simulink model "integrated_model"  (R2020b)
settings: Solver=VariableStepAuto  StartTime=0.0  StopTime=10  RelTol=1e-3
undefined symbols (not defined in the file): sigbuilder_block
settings Model: Creator=Training  LastModifiedBy=Training

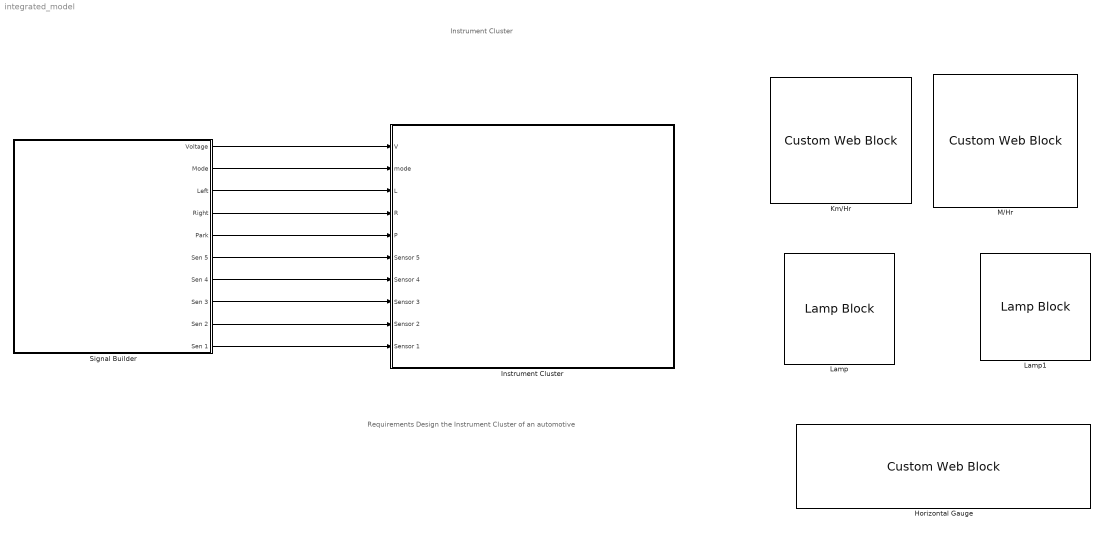
== system integrated_model ==
  note: Requirements
      | Design the Instrument Cluster of an automotive
  note: Instrument Cluster
  Horizontal Gauge : CustomWebBlock  ShowInitialText=on  Configuration="{\"components\":[{\"name\":\"LinearScaleComponent\",\"settings\":{\"bounds\":{\"max\":5,\"min\":0,\"tickInterval\":\"auto\"},\"internalTickHeightScaleFactor\":0.5,\"labelColor\":[250,245,199],\"labelFont\":{\"font\":\"Arial\",\"fontSize\":12},\"labelTransparency\":1,\"needleImage\":{\"size\":[21,75],\"src\":\"data:image\\/svg+xml;base64,PHN2ZyB4bWxucz0iaHR0cDovL3d3dy53My5vcmcvMjAwMC9zdmciIHhtbG5zOnhsaW5rPSJodHRwOi8vd3d3LnczLm9yZy8xOTk5L3hsaW5rIiB2aWV3Qm94PSIwIDAgMjEgNzUiPjxkZWZzPjxzdHlsZT4uY2xzLTF7ZmlsbDpub25lO30uY2xzLTJ7aXNvbGF0aW9uOmlzb2xhdGU7fS5jbHMtM3tjbGlwLXBhdGg6dXJsKCNjbGlwLXBhdGgpO30uY2xzLTR7b3BhY2l0eTowLjM7bWl4LWJsZW5kLW1vZGU6bXVsdGlwbHk7fS5jbHMtNXtmaWxsOiNlYjI2Mjk7fTwvc3R5bGU+PGNsaXBQYXRoIGlkPSJjbGlwLXBhdGgiIHRyYW5zZm9y ...(+1928 chars)\",\"srcOrientation\":\"horizontal\"},\"needleOffset\":[0,0.01094391244870041],\"needleSize\":{\"height\":0.7589285714285714,\"width\":0.11960078534031414},\"position\":[0.06986607142857143,0.01995798319327731,0.9641544117647058,0.8],\"scaleColors\":[],\"scaleColorsSize\":0.2,\"showLabels\":1,\"showMinorTicks\":0,\"showSpanLine\":1,\"showTicks\":1,\"tickColor\":[250,245,200],\"tickTransparency\":1,\"valueBarColor\":[23,89,176],\"valueBarOffset\":0,\"valueBarSize\":0.23,\"valueBarTransparency\":1}},{\"name\":\"BackgroundImageComponent\",\"settings\":{\"image\":{\"size\":[380,101],\"src\":\"data:image\\/svg+xml;base64,PHN2ZyB4bWxucz0iaHR0cDovL3d3dy53My5vcmcvMjAwMC9zdmciIHZpZXdCb3g9IjAgMCAzODAgMTAxIj48ZGVmcz48c3R5bGU+LmNscy0xe2ZpbGw6IzAwMmI0Mjt9LmNscy0ye2ZpbGw6IzQyNzA4Mjt9LmNscy0ze2ZpbGw6IzdjYTBiMjt9PC9zdHlsZT48L2RlZnM+PHRpdGxlPmhvcml6b250YWxfZ2F1Z2VfIGJhY2tncm91bmQ8L3RpdGxlPjxnIGlkPSJMYXllcl8yIiBkYXRhLW5hbWU9IkxheWVyIDIiPjxnIGlkPSJMYXllcl8xLTIiIGRhdGEtbmFtZT0iTGF5ZXIgMSI+PHJlY3QgY2xhc3M9ImNscy0xIiB4PSIxMSIgeT0iMTEiIHdpZHRoPSIzNTgiIGhlaWdodD0iNzkiLz48cGF0aCBjbGFzcz0iY2xzLTIiIGQ9Ik04LDhWOTNIMzcyVjhaTTM2OSw5MEgxMVYxMUgzNjlaIi8+PHBhdGggY2xhc3M9ImNscy0zIiBkPSJNMCwwVjEwMUgzODBWMFpNMzcyLDkzSDhWOEgzNzJaIi8+PC9nPjwvZz48L3N2Zz4=\",\"srcOrientation\":\"horizontal\"},\"position\":[0,0,1,1],\"scaleMode\":\"0\"}},{\"name\":\"ForegroundImageComponent\",\"settings\":{\"image\":{\"size\":[0,0],\"src\":\"default\",\"srcOrientation\":[]},\"isForeground\":1,\"position\":[0,0,1,1],\"scaleMode\":\"0\"}}],\"settings\":{\"BindingType\":\"signal\",\"aspectRatio\":3.8,\"fixedAspectRatio\":\"on\",\"orientation\":\"horizontal\"},\"type\":\"LinearGauge\"}"
  Instrument Cluster : Subsystem
  Km/Hr : CustomWebBlock  LabelPosition=Hide  ShowInitialText=on  Configuration="{\"components\":[{\"name\":\"CircularScaleComponent\",\"settings\":{\"bounds\":{\"max\":100,\"min\":0,\"tickInterval\":\"auto\"},\"direction\":\"cw\",\"flipLimits\":0,\"innerRadius\":0.75,\"internalTickHeightScaleFactor\":1,\"labelColor\":[255,252,199],\"labelFont\":{\"font\":\"Arial\",\"fontSize\":12},\"labelTransparency\":1,\"minorTickHeightScaleFactor\":0.2,\"needleImage\":{\"size\":[1890,567],\"src\":\"data:image\\/svg+xml;base64,PD94bWwgdmVyc2lvbj0iMS4wIiBlbmNvZGluZz0iVVRGLTgiIHN0YW5kYWxvbmU9Im5vIj8+CjxzdmcKICAgeG1sbnM6ZGM9Imh0dHA6Ly9wdXJsLm9yZy9kYy9lbGVtZW50cy8xLjEvIgogICB4bWxuczpjYz0iaHR0cDovL2NyZWF0aXZlY29tbW9ucy5vcmcvbnMjIgogICB4bWxuczpyZGY9Imh0dHA6Ly93d3cudzMub3JnLzE5OTkvMDIvMjItcmRmLXN5bnRheC1ucyMiCiAgIHhtbG5zOnN2Zz0iaHR0cDovL3d3dy53My5vcmcvMjAwMC9zdmciCiAgIHhtbG5zPSJodHRwOi8vd3d3LnczLm9yZy8yMDAwL3N2ZyIKICAgeG1sbnM6 ...(+4096 chars)\"},\"needleOffset\":[0.1610917094974375,0],\"needleOrientation\":-45,\"needleRotation\":180.59702388394928,\"needleSize\":{\"height\":0.13032601008944536,\"width\":0.416859542883425},\"outerRadius\":0.9,\"position\":[0.06486742424242424,0.05627705627705628,0.8917748917748918,0.8787878787878788],\"scaleAngle\":270,\"scaleAngleOffset\":135,\"scaleColors\":[],\"scaleColorsSize\":0.2,\"scalePosition\":[0,0,1,1],\"showLabels\":1,\"showMinorTicks\":1,\"showSpanLine\":1,\"showTicks\":1,\"tickColor\":[15,255,255],\"tickTransparency\":1,\"valueBarColor\":[19,159,255],\"valueBarPosition\":[0,0,1,1],\"valueBarSize\":0.2,\"valueBarTransparency\":1}},{\"name\":\"BackgroundImageComponent\",\"settings\":{\"image\":{\"size\":[500,500],\"src\":\"data:image\\/svg+xml;base64,PD94bWwgdmVyc2lvbj0iMS4wIiBlbmNvZGluZz0iVVRGLTgiIHN0YW5kYWxvbmU9Im5vIj8+CjxzdmcKICAgeG1sbnM6ZGM9Imh0dHA6Ly9wdXJsLm9yZy9kYy9lbGVtZW50cy8xLjEvIgogICB4bWxuczpjYz0iaHR0cDovL2NyZWF0aXZlY29tbW9ucy5vcmcvbnMjIgogICB4bWxuczpyZGY9Imh0dHA6Ly93d3cudzMub3JnLzE5OTkvMDIvMjItcmRmLXN5bnRheC1ucyMiCiAgIHhtbG5zOnN2Zz0iaHR0cDovL3d3dy53My5vcmcvMjAwMC9zdmciCiAgIHhtbG5zPSJodHRwOi8vd3d3LnczLm9yZy8yMDAwL3N2ZyIKICAgeG1sbnM6 ...(+9964 chars)\"},\"position\":[0,0,1,1],\"scaleMode\":\"0\"}},{\"name\":\"ForegroundImageComponent\",\"settings\":{\"image\":{\"size\":[0,0],\"src\":\"default\",\"srcOrientation\":[]},\"isForeground\":1,\"position\":[0,0,1,1],\"scaleMode\":\"0\"}}],\"settings\":{\"BindingType\":\"signal\",\"aspectRatio\":1.035294117647059,\"direction\":\"cw\",\"fixedAspectRatio\":\"on\",\"flipLimits\":0,\"orientation\":\"horizontal\"},\"type\":\"CircularGauge\"}"
  Lamp : LampBlock
  Lamp1 : LampBlock
  M/Hr : CustomWebBlock  LabelPosition=Hide  ShowInitialText=on  Configuration="{\"components\":[{\"name\":\"CircularScaleComponent\",\"settings\":{\"bounds\":{\"max\":100,\"min\":0,\"tickInterval\":\"auto\"},\"direction\":\"cw\",\"flipLimits\":0,\"innerRadius\":0.75,\"internalTickHeightScaleFactor\":1,\"labelColor\":[0,114,189],\"labelFont\":{\"font\":\"Arial\",\"fontSize\":12},\"labelTransparency\":1,\"minorTickHeightScaleFactor\":0.2,\"needleImage\":{\"size\":[1890,567],\"src\":\"data:image\\/svg+xml;base64,PD94bWwgdmVyc2lvbj0iMS4wIiBlbmNvZGluZz0iVVRGLTgiIHN0YW5kYWxvbmU9Im5vIj8+CjxzdmcKICAgeG1sbnM6ZGM9Imh0dHA6Ly9wdXJsLm9yZy9kYy9lbGVtZW50cy8xLjEvIgogICB4bWxuczpjYz0iaHR0cDovL2NyZWF0aXZlY29tbW9ucy5vcmcvbnMjIgogICB4bWxuczpyZGY9Imh0dHA6Ly93d3cudzMub3JnLzE5OTkvMDIvMjItcmRmLXN5bnRheC1ucyMiCiAgIHhtbG5zOnN2Zz0iaHR0cDovL3d3dy53My5vcmcvMjAwMC9zdmciCiAgIHhtbG5zPSJodHRwOi8vd3d3LnczLm9yZy8yMDAwL3N2ZyIKICAgeG1sbnM6 ...(+4096 chars)\"},\"needleOffset\":[0.1610917094974375,0],\"needleOrientation\":-45,\"needleRotation\":180.59702388394928,\"needleSize\":{\"height\":0.13032601008944536,\"width\":0.416859542883425},\"outerRadius\":0.9,\"position\":[0.06475601604278075,0.05626539408866995,0.8917795566502463,0.8787600267379679],\"scaleAngle\":270,\"scaleAngleOffset\":135,\"scaleColors\":[],\"scaleColorsSize\":0.2,\"scalePosition\":[0,0,1,1],\"showLabels\":1,\"showMinorTicks\":1,\"showSpanLine\":1,\"showTicks\":1,\"tickColor\":[100,212,19],\"tickTransparency\":1,\"valueBarColor\":[0,114,189],\"valueBarPosition\":[0,0,1,1],\"valueBarSize\":0.2,\"valueBarTransparency\":1}},{\"name\":\"BackgroundImageComponent\",\"settings\":{\"image\":{\"size\":[500,500],\"src\":\"data:image\\/svg+xml;base64,PD94bWwgdmVyc2lvbj0iMS4wIiBlbmNvZGluZz0iVVRGLTgiIHN0YW5kYWxvbmU9Im5vIj8+CjxzdmcKICAgeG1sbnM6ZGM9Imh0dHA6Ly9wdXJsLm9yZy9kYy9lbGVtZW50cy8xLjEvIgogICB4bWxuczpjYz0iaHR0cDovL2NyZWF0aXZlY29tbW9ucy5vcmcvbnMjIgogICB4bWxuczpyZGY9Imh0dHA6Ly93d3cudzMub3JnLzE5OTkvMDIvMjItcmRmLXN5bnRheC1ucyMiCiAgIHhtbG5zOnN2Zz0iaHR0cDovL3d3dy53My5vcmcvMjAwMC9zdmciCiAgIHhtbG5zPSJodHRwOi8vd3d3LnczLm9yZy8yMDAwL3N2ZyIKICAgeG1sbnM6 ...(+9964 chars)\"},\"position\":[0,0,1,1],\"scaleMode\":\"0\"}},{\"name\":\"ForegroundImageComponent\",\"settings\":{\"image\":{\"size\":[0,0],\"src\":\"default\",\"srcOrientation\":[]},\"isForeground\":1,\"position\":[0,0,1,1],\"scaleMode\":\"0\"}}],\"settings\":{\"BindingType\":\"signal\",\"aspectRatio\":1.085561497326203,\"direction\":\"cw\",\"fixedAspectRatio\":\"on\",\"flipLimits\":0,\"orientation\":\"horizontal\"},\"type\":\"CircularGauge\"}"
  Signal Builder : Subsystem  Tag=STV Subsys  LoadFcn=sigbuilder_block('load');  StartFcn=sigbuilder_block('start');  StopFcn=sigbuilder_block('stop');  ClipboardFcn=sigbuilder_block('clipboard');  mask(Sigbuilder block){tuvar=[0:10]}
      mask help: Simulink:masks:SigbuilderBlock_MD
      mask init:
      | if ~strcmp(get_param(bdroot(gcbh),'SimulationStatus'),'stopped') tuvar = sigbuilder_block('maskInit'); end
      settings: CopyFcn=sigbuilder_block('copy');  DeleteFcn=sigbuilder_block('delete');  ModelCloseFcn=sigbuilder_block('modelClose');  PreSaveFcn=sigbuilder_block('preSave');  PauseFcn=sigbuilder_block('pause');  ContinueFcn=sigbuilder_block('continue');  NameChangeFcn=sigbuilder_block('namechange');  OpenFcn=sigbuilder_block('open',[539.25 204.75 550.5 399.75 ]);  CloseFcn=sigbuilder_block('close');
      mask Display: plot(0, 0, 100, 100,[2, 2, 32, 32, 2], [68, 8, 8, 68, 68],[32, 2], [38, 38], [32, 19, 2],[53, 60, 44], [32, 17, 17, 2],[16, 16, 31, 31]);txt = getActiveGroup(gcbh);text(2, 100, txt,'verticalAlignment', 'top');
  wires:
  Signal Builder/1(Voltage) -> Instrument Cluster/1(V)
  Signal Builder/2(Mode) -> Instrument Cluster/2(mode)
  Signal Builder/3(Left) -> Instrument Cluster/3(L)
  Signal Builder/4(Right) -> Instrument Cluster/4(R)
  Signal Builder/5(Park) -> Instrument Cluster/5(P)
  Signal Builder/6("Sen 5 ") -> Instrument Cluster/6(Sensor 5)
  Signal Builder/7(Sen 4) -> Instrument Cluster/7(Sensor 4)
  Signal Builder/8(Sen 3) -> Instrument Cluster/8(Sensor 3)
  Signal Builder/9(" Sen 2") -> Instrument Cluster/9(Sensor 2)
  Signal Builder/10(Sen 1) -> Instrument Cluster/10(Sensor 1)

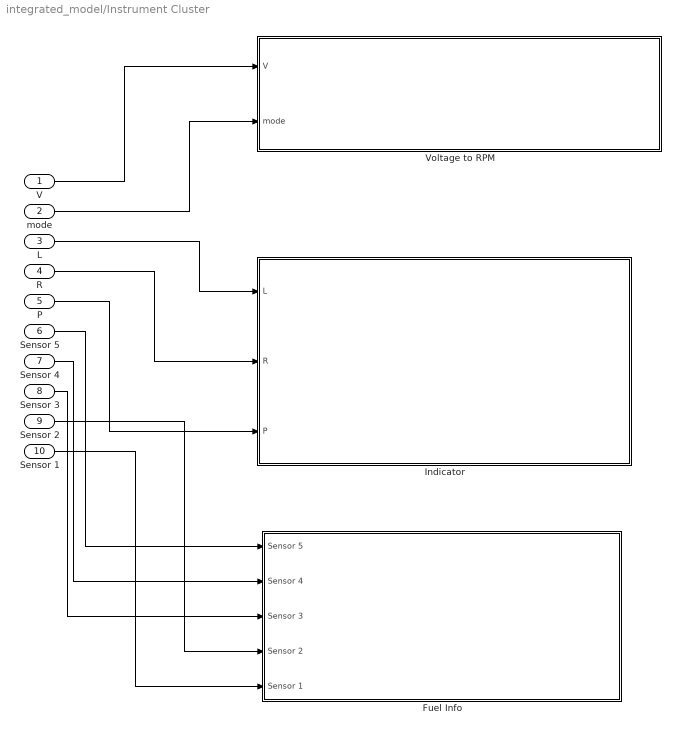
== system integrated_model/Instrument Cluster ==
  V : Inport
  mode : Inport  Port=2
  L : Inport  Port=3
  R : Inport  Port=4
  P : Inport  Port=5
  Sensor 5 : Inport  Port=6
  Sensor 4 : Inport  Port=7
  Sensor 3 : Inport  Port=8
  Sensor 2 : Inport  Port=9
  Sensor 1 : Inport  Port=10
  Fuel Info : Subsystem
  Indicator : Subsystem
  Voltage to RPM : Subsystem
  wires:
  mode/1 -> Voltage to RPM/2(mode)
  Sensor 3/1 -> Fuel Info/3(Sensor 3)
  V/1 -> Voltage to RPM/1(V)
  R/1 -> Indicator/2(R)
  Sensor 4/1 -> Fuel Info/2(Sensor 4)
  Sensor 5/1 -> Fuel Info/1(Sensor 5)
  P/1 -> Indicator/3(P)
  Sensor 2/1 -> Fuel Info/4(Sensor 2)
  L/1 -> Indicator/1(L)
  Sensor 1/1 -> Fuel Info/5(Sensor 1)

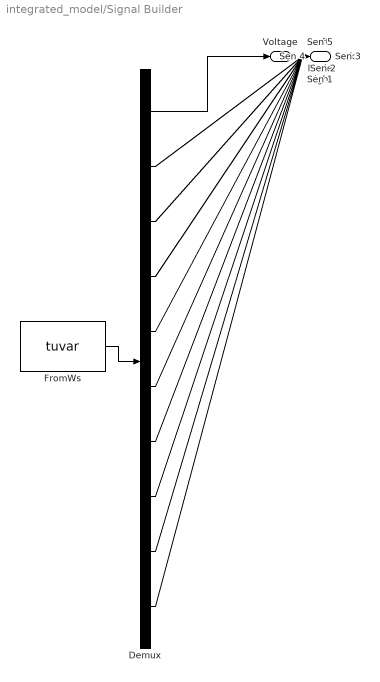
== system integrated_model/Signal Builder ==
  Demux : Demux  Tag=STV Demux  Outputs=10
      settings: DisplayOption=none
  FromWs : FromWorkspace  Tag=STV FromWs  VariableName=tuvar
      SigBuilderData=|
      | common.afterFinalStr = 'Extrapolate'
      | common.sampleTime = 0
      | dataSet.timeRange = [0 10]
      | dataSet.name = 'Group 1'
      | sbobj.Groups.Name = 'Group 1'
      | sbobj.Groups.Signals(1).Name = 'Voltage'
      | sbobj.Groups.Signals(1).XData = [0 1 2 3 4 5 6 7 8 9 10]
      | sbobj.Groups.Signals(1).YData = [5 5 4 5 8 6 4 7 1 2 9]
      | sbobj.Groups.Signals(2).Name = 'Mode'
      | sbobj.Groups.Signals(2).XData = [0 2 3 4 5 6 7 8 9 10]
      | sbobj.Groups.Signals(2).YData = [1 1 1 0 0 1 0 1 0 1]
      | sbobj.Groups.Signals(3).Name = 'Left'
      | sbobj.Groups.Signals(3).XData = [0 2 3 4 5 6 7 8 9 10]
      | sbobj.Groups.Signals(3).YData = [0 0 0 1 1 1 1 1 0 0]
      | sbobj.Groups.Signals(4).Name = 'Right'
      | sbobj.Groups.Signals(4).XData = [0 1 2 3 4 5 6 7 8 9 10]
      | sbobj.Groups.Signals(4).YData = [0 0 1 1 0 0 0 0 0 0 0]
      | sbobj.Groups.Signals(5).Name = 'Park'
      | sbobj.Groups.Signals(5).XData = [0 1 2 3 4 5 6 7 8 9 10]
      | sbobj.Groups.Signals(5).YData = [1 1 0 0 0 0 0 0 0 1 1]
      | sbobj.Groups.Signals(6).Name = 'Sen 5 '
      | sbobj.Groups.Signals(6).XData = [0 2 3 4 5 6 7 8 9 10]
      | sbobj.Groups.Signals(6).YData = [0 0 0 0 0 1 0 0 0 1]
      | sbobj.Groups.Signals(7).Name = 'Sen 4'
      | sbobj.Groups.Signals(7).XData = [0 2 3 4 5 6 7 8 9 10]
      | sbobj.Groups.Signals(7).YData = [0 0 0 1 0 1 0 1 0 1]
      | sbobj.Groups.Signals(8).Name = 'Sen 3'
      | sbobj.Groups.Signals(8).XData = [0 1 2 3 4 5 6 7 8 9 10]
      | sbobj.Groups.Signals(8).YData = [1 1 0 1 1 0 1 0 1 1 1]
      | sbobj.Groups.Signals(9).Name = ' Sen 2'
      | sbobj.Groups.Signals(9).XData = [0 2 3 4 5 6 7 8 9 10]
      | sbobj.Groups.Signals(9).YData = [1 1 1 1 0 1 0 1 1 1]
      | sbobj.Groups.Signals(10).Name = 'Sen 1'
      | sbobj.Groups.Signals(10).XData = [0 2 3 4 5 6 7 8 9 10]
      | sbobj.Groups.Signals(10).YData = [1 1 1 1 1 1 1 1 1 1]
  Voltage : Outport  Tag=STV Outport
  Mode : Outport  Tag=STV Outport  Port=2
  Left : Outport  Tag=STV Outport  Port=3
  Right : Outport  Tag=STV Outport  Port=4
  Park : Outport  Tag=STV Outport  Port=5
  "Sen 5 " : Outport  Tag=STV Outport  Port=6
  Sen 4 : Outport  Tag=STV Outport  Port=7
  Sen 3 : Outport  Tag=STV Outport  Port=8
  " Sen 2" : Outport  Tag=STV Outport  Port=9
  Sen 1 : Outport  Tag=STV Outport  Port=10
  wires:
  FromWs/1 -> Demux/1
  Demux/1 -> Voltage/1
  Demux/2 -> Mode/1
  Demux/3 -> Left/1
  Demux/4 -> Right/1
  Demux/5 -> Park/1
  Demux/6 -> "Sen 5 "/1
  Demux/7 -> Sen 4/1
  Demux/8 -> Sen 3/1
  Demux/9 -> " Sen 2"/1
  Demux/10 -> Sen 1/1

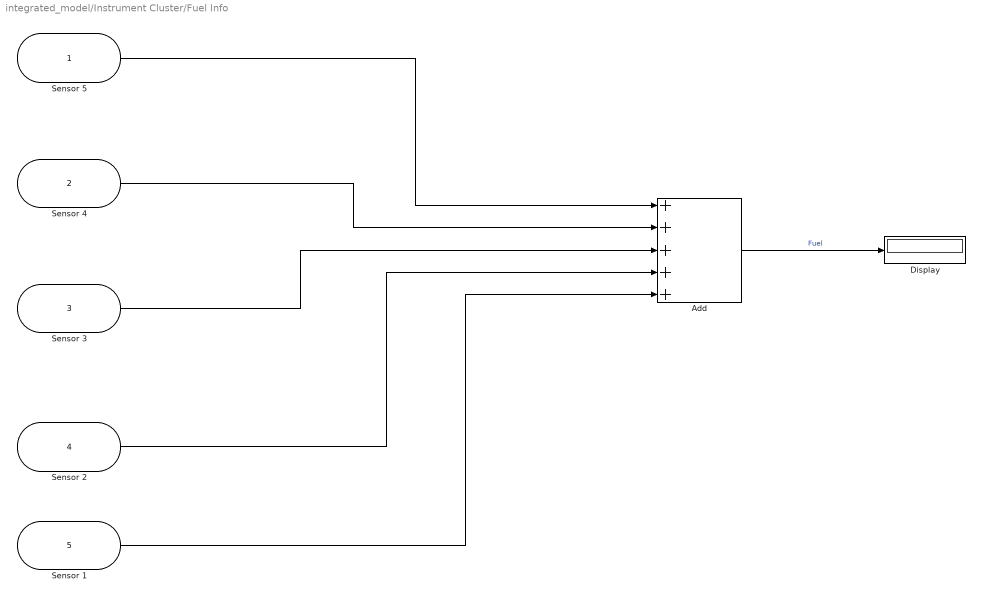
== system integrated_model/Instrument Cluster/Fuel Info ==
  Sensor 5 : Inport
  Sensor 4 : Inport  Port=2
  Sensor 3 : Inport  Port=3
  Sensor 2 : Inport  Port=4
  Sensor 1 : Inport  Port=5
  Add : Sum  Inputs=+++++
  Display : Display
  wires:
  Add/1 -> Display/1  "Fuel"
  Sensor 4/1 -> Add/2
  Sensor 1/1 -> Add/5
  Sensor 3/1 -> Add/3
  Sensor 5/1 -> Add/1
  Sensor 2/1 -> Add/4

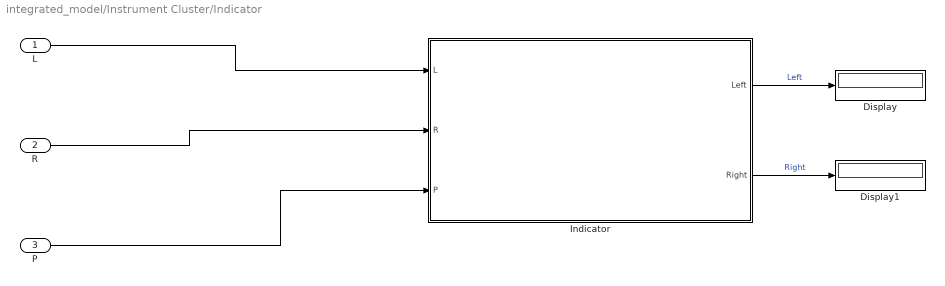
== system integrated_model/Instrument Cluster/Indicator ==
  L : Inport
  R : Inport  Port=2
  P : Inport  Port=3
  Display : Display
  Display1 : Display
  Indicator : Subsystem
  wires:
  L/1 -> Indicator/1(L)
  Indicator/1(Left) -> Display/1  "Left"
  Indicator/2(Right) -> Display1/1  "Right"
  P/1 -> Indicator/3(P)
  R/1 -> Indicator/2(R)

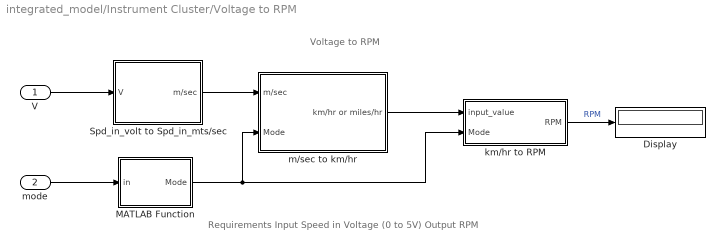
== system integrated_model/Instrument Cluster/Voltage to RPM ==
  note: Requirements
      | Input
      | Speed in Voltage (0 to 5V)
      | Output
      | RPM
  note: Voltage to RPM
  V : Inport
  mode : Inport  Port=2
  Display : Display
  MATLAB Function : MATLAB Function  TreatAsAtomicUnit=on
  Spd_in_volt to Spd_in_mts/sec : Subsystem
  km/hr to RPM : Subsystem  mask{inch=28}
      mask prompts: inch "Enter the wheel dameter in inches"
  m/sec to km/hr : Subsystem
  wires:
  mode/1 -> MATLAB Function/1(in)
  MATLAB Function/1(Mode) -> km/hr to RPM/2(Mode), m/sec to km/hr/2(Mode)
  V/1 -> Spd_in_volt to Spd_in_mts/sec/1(V)
  km/hr to RPM/1(RPM) -> Display/1  "RPM"
  m/sec to km/hr/1("km/hr or miles/hr ") -> km/hr to RPM/1(input_value)
  Spd_in_volt to Spd_in_mts/sec/1("m/sec ") -> m/sec to km/hr/1(m/sec)

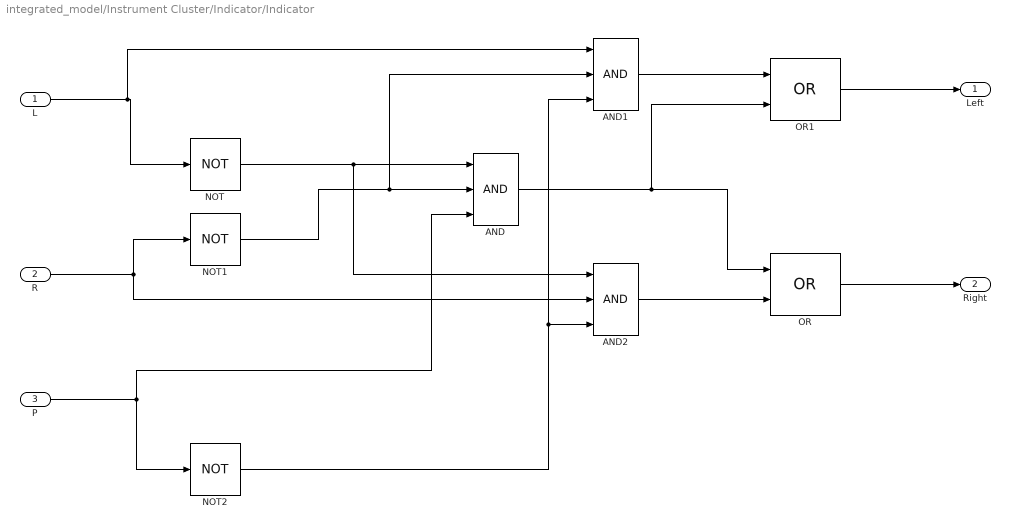
== system integrated_model/Instrument Cluster/Indicator/Indicator ==
  L : Inport
  R : Inport  Port=2
  P : Inport  Port=3
  AND : Logic  Inputs=3  IconShape=distinctive  AllPortsSameDT=off  OutDataTypeStr=boolean
  AND1 : Logic  Inputs=3  IconShape=distinctive  AllPortsSameDT=off  OutDataTypeStr=boolean
  AND2 : Logic  Inputs=3  IconShape=distinctive  AllPortsSameDT=off  OutDataTypeStr=boolean
  NOT : Logic  Operator=NOT  IconShape=distinctive  AllPortsSameDT=off  OutDataTypeStr=boolean
  NOT1 : Logic  Operator=NOT  IconShape=distinctive  AllPortsSameDT=off  OutDataTypeStr=boolean
  NOT2 : Logic  Operator=NOT  IconShape=distinctive  AllPortsSameDT=off  OutDataTypeStr=boolean
  OR : Logic  Operator=OR  IconShape=distinctive  AllPortsSameDT=off  OutDataTypeStr=boolean
  OR1 : Logic  Operator=OR  IconShape=distinctive  AllPortsSameDT=off  OutDataTypeStr=boolean
  Left : Outport
  Right : Outport  Port=2
  wires:
  OR/1 -> Right/1
  R/1 -> AND2/2, NOT1/1
  NOT1/1 -> AND1/2, AND/2
  NOT/1 -> AND2/1, AND/1
  AND2/1 -> OR/2
  NOT2/1 -> AND1/3, AND2/3
  AND1/1 -> OR1/1
  AND/1 -> OR1/2, OR/1
  P/1 -> NOT2/1, AND/3
  L/1 -> AND1/1, NOT/1
  OR1/1 -> Left/1

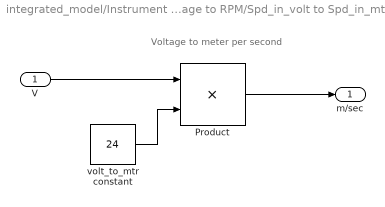
== system integrated_model/Instrument Cluster/Voltage to RPM/Spd_in_volt to Spd_in_mts//sec ==
  note: Voltage to meter per second
  V : Inport
  Product : Product
  volt_to_mtr constant : Constant  Value=24
  "m/sec " : Outport
  wires:
  Product/1 -> "m/sec "/1
  volt_to_mtr constant/1 -> Product/2
  V/1 -> Product/1

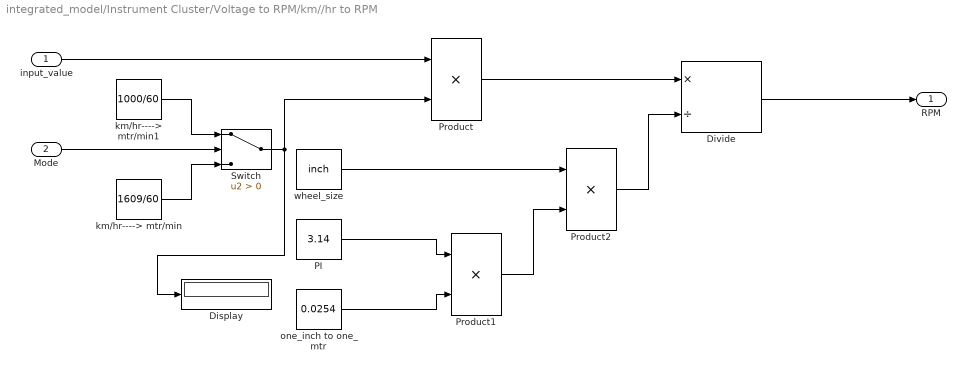
== system integrated_model/Instrument Cluster/Voltage to RPM/km//hr to RPM ==
  input_value : Inport
  Mode : Inport  Port=2
  Display : Display
  Divide : Product  Inputs=*/
  PI : Constant  Value=3.14
  Product : Product
  Product1 : Product
  Product2 : Product
  Switch : Switch  Criteria=u2 > Threshold
  km/hr----> mtr/min : Constant  Value=1609/60
  km/hr----> mtr/min1 : Constant  Value=1000/60
  one_inch to one_mtr : Constant  Value=0.0254
  wheel_size : Constant  Value=inch
  RPM : Outport
  wires:
  one_inch to one_mtr/1 -> Product1/2
  PI/1 -> Product1/1
  wheel_size/1 -> Product2/1
  Product1/1 -> Product2/2
  Product/1 -> Divide/1
  Product2/1 -> Divide/2
  Divide/1 -> RPM/1
  input_value/1 -> Product/1
  km/hr----> mtr/min1/1 -> Switch/1
  km/hr----> mtr/min/1 -> Switch/3
  Mode/1 -> Switch/2
  Switch/1 -> Product/2, Display/1

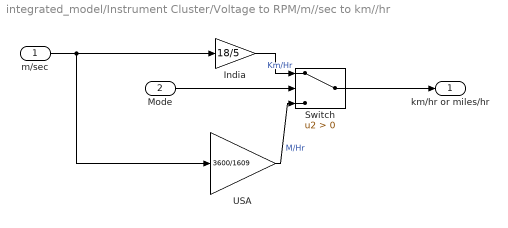
== system integrated_model/Instrument Cluster/Voltage to RPM/m//sec to km//hr ==
  m/sec : Inport
  Mode : Inport  Port=2
  India : Gain  Gain=18/5
  Switch : Switch  Criteria=u2 > Threshold
  USA : Gain  Gain=3600/1609
  "km/hr or miles/hr " : Outport
  wires:
  m/sec/1 -> USA/1, India/1
  India/1 -> Switch/1  "Km/Hr"
  Switch/1 -> "km/hr or miles/hr "/1
  Mode/1 -> Switch/2
  USA/1 -> Switch/3  "M/Hr"

== matlab function integrated_model/Instrument Cluster/Voltage to RPM/MATLAB Function ==
  data: in input; Mode output
function Mode = Modeselect(in)
    if(in==0)
        Mode=0; % m/sec is converted to miles/hr
    else
        Mode=1; % m/sec is converted to km/hr
    end
